simulink model "SystemSISOC"  (R2022b)
settings: Solver=ode45  StartTime=0.0  StopTime=tend  MaxStep=0.01  RelTol=1e-3  EnableMultiTasking=on
values from neighbouring files (symbols this model uses):
  sigma2e = 0.1    [L3_ocet_init.m]
  Tf = 8*Tp    (= 0.4)    [L3_ocet_init.m]
  Tp = 0.1    [L1_dzban_Init.m]    (also in L2_czolg_init.m; L3_ocet_init.m = 0.05)
libraries: simulink x1
settings Model: Creator=molsz  LastModifiedBy=molsz
settings SolverCC: AlgebraicLoopSolver=TrustRegion
settings DataIOCC: LimitDataPoints=on  SaveFormat=Array  SignalLoggingSaveFormat=ModelDataLogs  ReturnWorkspaceOutputs=off
settings OptimizationCC: InitFltsAndDblsToZero=on  LifeSpan=inf
settings DebuggingCC: SaveWithParameterizedLinksMsg=none  UnderspecifiedInitializationDetection=Classic  MergeDetectMultiDrivingBlocksExec=none  SignalResolutionControl=TryResolveAllWithWarning  SolverPrmCheckMsg=warning  MultiTaskDSMMsg=warning  MultiTaskCondExecSysMsg=none  FcnCallInpInsideContextMsg=warning  UnconnectedInputMsg=warning  UnconnectedOutputMsg=warning  UnconnectedLineMsg=warning  SFUnexpectedBacktrackingDiag=warning  SFNoUnconditionalDefaultTransitionDiag=warning  SFExecutionAtInitializationDiag=none  SFMachineParentedDataDiag=warning  ArithmeticOperatorsInVariantConditions=warning
settings HardwareCC: ProdBitPerPointer=32  ProdBitPerSizeT=32  ProdBitPerPtrDiffT=32  ProdLargestAtomicFloat=None  ProdIntDivRoundTo=Undefined  ProdEndianess=Unspecified  ProdWordSize=32  ProdHWDeviceType=32-bit Generic
settings ModelReferenceCC: PropagateSignalLabelsOutOfModel=off
settings CodeAppCC: StateflowObjectComments=on
settings GRTTargetCC: TargetFcnLib=ansi_tfl_tmw.mat  TargetLangStandard=C89/C90 (ANSI)  CombineOutputUpdateFcns=off  GRTInterface=on
settings ConfigComp: CovMetricSettings=dw  CovSaveCumulativeToWorkspaceVar=on  CovSaveSingleToWorkspaceVar=on

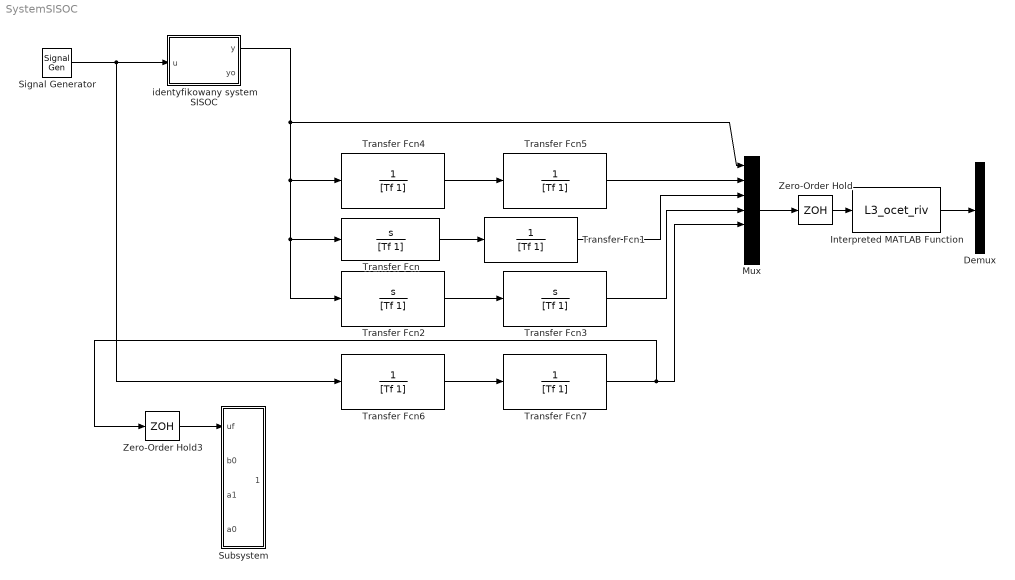
== system SystemSISOC ==
  Demux : Demux
  Interpreted MATLAB Function : MATLABFcn  MATLABFcn=L3_ocet_riv  OutputDimensions=4
  Mux : Mux  Inputs=7
  Signal Generator : SignalGenerator  WaveForm=square  Frequency=0.04
  Subsystem : Subsystem
  Transfer Fcn : TransferFcn  Numerator=[1 0]  Denominator=[Tf 1]
  Transfer Fcn{1,4..7} (5 alike) : TransferFcn  Denominator=[Tf 1]
  Transfer Fcn2 : TransferFcn  Numerator=[1 0]  Denominator=[Tf 1]
  Transfer Fcn3 : TransferFcn  Numerator=[1 0]  Denominator=[Tf 1]
  Zero-Order Hold : ZeroOrderHold  SampleTime=Tp
  Zero-Order Hold3 : ZeroOrderHold  SampleTime=Tp
  identyfikowany system SISOC : Subsystem
  wires:
  Signal Generator/1 -> Transfer Fcn6/1, identyfikowany system SISOC/1(u)
  Transfer Fcn/1 -> Transfer Fcn1/1
  Transfer Fcn2/1 -> Transfer Fcn3/1
  identyfikowany system SISOC/1(y) -> Transfer Fcn4/1, Transfer Fcn/1, Transfer Fcn2/1, Mux/1
  Transfer Fcn1/1 -> Mux/3
  Transfer Fcn3/1 -> Mux/4
  Transfer Fcn5/1 -> Mux/2
  Transfer Fcn4/1 -> Transfer Fcn5/1
  Transfer Fcn6/1 -> Transfer Fcn7/1
  Transfer Fcn7/1 -> Zero-Order Hold3/1, Mux/5
  Zero-Order Hold3/1 -> Subsystem/1(uf)
  Mux/1 -> Zero-Order Hold/1
  Zero-Order Hold/1 -> Interpreted MATLAB Function/1
  Interpreted MATLAB Function/1 -> Demux/1

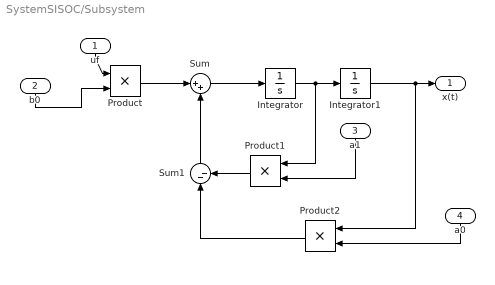
== system SystemSISOC/Subsystem ==
  uf : Inport
  "b0 " : Inport  Port=2
  a1 : Inport  Port=3
  a0 : Inport  Port=4
  Integrator : Integrator
  Integrator1 : Integrator
  Product : Product  RndMeth=Zero  SampleTime=Tp
  Product1 : Product  RndMeth=Zero  SampleTime=Tp
  Product2 : Product  RndMeth=Zero  SampleTime=Tp
  Sum : Sum  Inputs=|++  SampleTime=Tp
  Sum1 : Sum  Inputs=|--  SampleTime=Tp
  x(t) : Outport  VectorParamsAs1DForOutWhenUnconnected=off
  wires:
  Product/1 -> Sum/1
  Sum/1 -> Integrator/1
  Integrator/1 -> Integrator1/1, Product1/1
  Integrator1/1 -> x(t)/1, Product2/1
  Sum1/1 -> Sum/2
  Product1/1 -> Sum1/2
  Product2/1 -> Sum1/1
  a0/1 -> Product2/2
  uf/1 -> Product/1
  "b0 "/1 -> Product/2
  a1/1 -> Product1/2

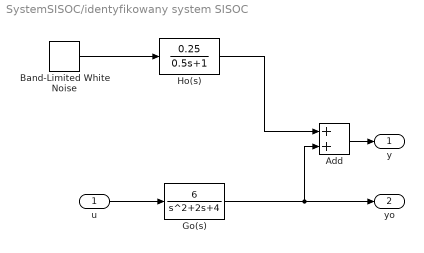
== system SystemSISOC/identyfikowany system SISOC ==
  u : Inport
  Add : Sum
  Band-Limited White Noise : simulink/Sources/Band-Limited White Noise  Cov=[sigma2e]  Ts=Tp*0.1  seed=[2941]
  Go(s) : TransferFcn  Numerator=[6]  Denominator=[1 2 4]
  Ho(s) : TransferFcn  Numerator=[0.25]  Denominator=[0.5 1]
  y : Outport
  yo : Outport  Port=2
  wires:
  Band-Limited White Noise/1 -> Ho(s)/1
  Ho(s)/1 -> Add/1
  Go(s)/1 -> Add/2, yo/1
  Add/1 -> y/1
  u/1 -> Go(s)/1
